simulink model "soft_control"  (R2020b)
settings: Solver=ode1be  StartTime=0.0  StopTime=inf  FixedStep=.01  RelTol=1e-3  EnableMultiTasking=on
undefined symbols (not defined in the file): deg, s
libraries: qbmove_library x4, dspmtrx3 x2, CP_library x1, QB_pacer_lib x1
settings Model: Creator=laurentio  LastModifiedBy=luca
settings DataIOCC: LimitDataPoints=on  SaveFormat=Array  ReturnWorkspaceOutputs=off
settings OptimizationCC: LifeSpan=inf
settings DebuggingCC: UnderspecifiedInitializationDetection=Classic  MergeDetectMultiDrivingBlocksExec=none  SolverPrmCheckMsg=warning  AllowSymbolicDim=off  StateNameClashWarn=warning  SFUnexpectedBacktrackingDiag=warning  SFNoUnconditionalDefaultTransitionDiag=warning  SFExecutionAtInitializationDiag=none  ArithmeticOperatorsInVariantConditions=warning
settings HardwareCC: ProdBitPerPointer=32  ProdBitPerSizeT=32  ProdBitPerPtrDiffT=32  ProdLargestAtomicFloat=None  ProdIntDivRoundTo=Undefined  ProdEndianess=Unspecified  ProdWordSize=32  ProdHWDeviceType=32-bit Generic
settings ModelReferenceCC: PropagateSignalLabelsOutOfModel=off
settings SFSimCC: SimUseLocalCustomCode=off  CustomCodeUndefinedFunction=UseInterfaceOnly
settings RTWCC: RTWUseLocalCustomCode=off
settings CodeAppCC: StateflowObjectComments=on
settings GRTTargetCC: TargetLangStandard=C89/C90 (ANSI)
settings ConfigComp: CovMetricSettings=dw  CovSaveCumulativeToWorkspaceVar=on  CovSaveSingleToWorkspaceVar=on  CovExternalEMLEnable=off  CovSFcnEnable=off

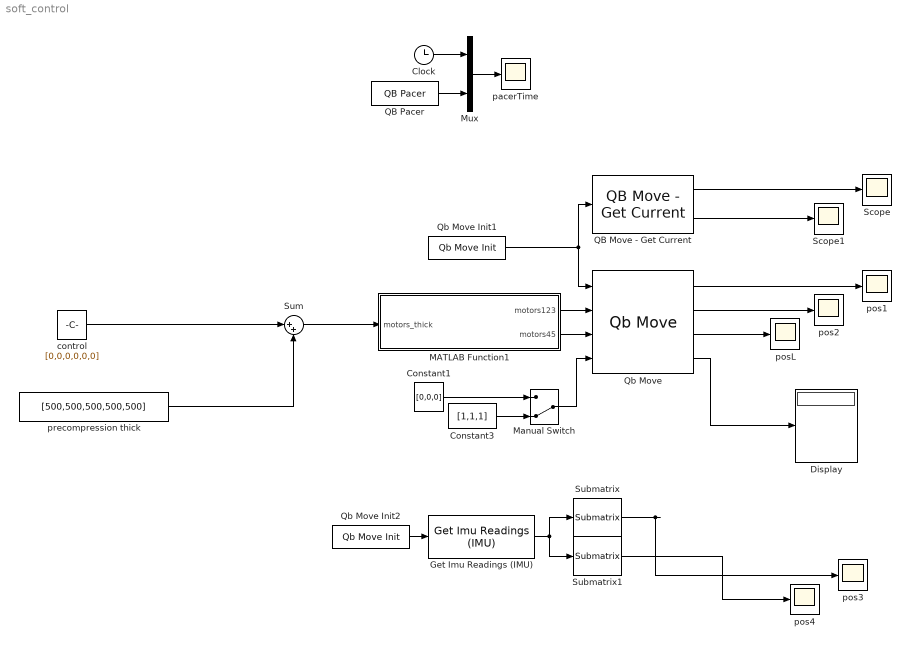
== system soft_control ==
  Clock : Clock
  Constant1 : Constant  Value=[0,0,0]
  Constant3 : Constant  Value=[1,1,1]
  Display : Display
  Get Imu Readings (IMU) : CP_library/Get Imu Readings (IMU)  ID=1  N_IMU=1  DAISY_CHAINING=off  ACC_UNITY=G  GYRO_UNITY=deg/s  MAG_UNITY=uT
      settings: SourceProductName=Centro Piaggio Library
  MATLAB Function1 : MATLAB Function  TreatAsAtomicUnit=on
  Manual Switch : ManualSwitch  CurrentSetting=0
  Mux : Mux  Inputs=2
  QB Move - Get Current : qbmove_library/QB Move - Get Current  ID=65  CONTROL_MODE=Prime Movers Positions  DAISY_CHAINING=off
      settings: SourceProductName=Qb Move Library
  QB Pacer : QB_pacer_lib/QB Pacer  simTimePerRealTime=1
      settings: SourceProductName=QB Pacer
  Qb Move : qbmove_library/Qb Move  ID=[1,2,3]  ACTIVE_COMM_DIRECTIONS=Both  CONTROL_MODE=Prime Movers Positions  DAISY_CHAINING=off  MAX_ANG=0  SW_LIMIT=inf  OFFSET=0  ACTIVATE=off  WDT=0.0  UNIT=TICK
      settings: SourceProductName=Qb Move Library
  Qb Move Init1 : qbmove_library/Qb Move Init  NUMBER_OF_COM='COM6'  BAUD_RATE_COM=2000000
      settings: SourceProductName=Qb Move Library
  Qb Move Init2 : qbmove_library/Qb Move Init  NUMBER_OF_COM='/dev/tty.usbserial-001'  BAUD_RATE_COM=2000000
      settings: SourceProductName=Qb Move Library
  Scope : Scope
  Scope1 : Scope
  Submatrix : dspmtrx3/Submatrix  RowSpan=Range of rows  RowStartMode=First  RowStartIndex=1  RowEndMode=Last  RowEndIndex=1  ColSpan=Range of columns  ColStartMode=Index  ColStartIndex=1  ColEndMode=Index  ColEndIndex=3
      settings: SourceProductBaseCode=SL
  Submatrix1 : dspmtrx3/Submatrix  RowSpan=Range of rows  RowStartMode=First  RowStartIndex=1  RowEndMode=Last  RowEndIndex=1  ColSpan=Range of columns  ColStartMode=Index  ColStartIndex=4  ColEndMode=Index  ColEndIndex=6
      settings: SourceProductBaseCode=SL
  Sum : Sum  Inputs=|++
  control : Constant  Value=[0,0,0,0,0,0]
  pacerTime : Scope
  pos{1..4} (4 alike) : Scope
  posL : Scope
  precompression thick : Constant  Value=[500,500,500,500,500]
  wires:
  QB Pacer/1 -> Mux/2
  Clock/1 -> Mux/1
  Constant1/1 -> Manual Switch/1
  Constant3/1 -> Manual Switch/2
  Qb Move/4 -> Display/1
  Mux/1 -> pacerTime/1
  Manual Switch/1 -> Qb Move/4
  Qb Move/1 -> pos1/1
  Qb Move/2 -> pos2/1
  Qb Move/3 -> posL/1
  Qb Move Init1/1 -> QB Move - Get Current/1, Qb Move/1
  QB Move - Get Current/1 -> Scope/1
  QB Move - Get Current/2 -> Scope1/1
  MATLAB Function1/1(motors123) -> Qb Move/2
  MATLAB Function1/2(motors45) -> Qb Move/3
  Sum/1 -> MATLAB Function1/1(motors_thick)
  precompression thick/1 -> Sum/2
  control/1 -> Sum/1
  Qb Move Init2/1 -> Get Imu Readings (IMU)/1
  Get Imu Readings (IMU)/1 -> Submatrix1/1, Submatrix/1
  Submatrix/1 -> pos3/1
  Submatrix1/1 -> pos4/1

== matlab function soft_control/MATLAB Function1 ==
  data: motors_thick input; motors123 output; motors45 output
function [motors123,motors45] = motor_remap(motors_thick)
    motors123(1) = motors_thick(1);
    motors123(2) = motors_thick(2);
    motors123(3) = motors_thick(3);
    motors45(1) = - motors_thick(4);
    motors45(2) = - motors_thick(5);
    motors45(3) = 0;
